simulink model "RobotResRateAlg"  (Simulink 7.8)
settings: Solver=ode45  StartTime=0.0  StopTime=simtime  RelTol=1e-3
values from neighbouring files (symbols this model uses):
  amp_C = 0.02    [projectCircle.m]
  freq_C = 2*pi/period    (= 0.1)    [projectCircle.m]
  Theta0 = fsolve(@inkinematic1,X0,optimset('Display','off'))    [projectCircle.m]
  Vx = 0    [projectCircle.m]
settings Model: Creator=carlossilvestre  LastModifiedBy=Administrator
settings DebuggingCC: SaveWithParameterizedLinksMsg=none  MultiTaskDSMMsg=warning  MultiTaskCondExecSysMsg=none  StrictBusMsg=None
settings RTWCC: IncludeERTFirstTime=on

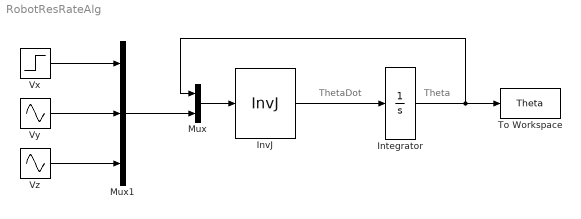
== system RobotResRateAlg ==
  note: ThetaDot
  note: Theta
  " Vz" : Sin  Amplitude=amp_C  Frequency=freq_C  Phase=pi/2  VectorParams1D=off
  Integrator : Integrator  InitialCondition=Theta0
  InvJ : MATLABFcn  MATLABFcn=InvJ  OutputDimensions=3
  Mux : Mux  Inputs=2
  Mux1 : Mux  Inputs=3
  To Workspace : ToWorkspace  VariableName=Theta  SampleTime=0.0342  SaveFormat=Array
  Vx : Step  Time=1000  Before=Vx  After=Vx
  Vy : Sin  Amplitude=amp_C  Frequency=freq_C  VectorParams1D=off
  wires:
  InvJ/1 -> Integrator/1
  Integrator/1 -> To Workspace/1, Mux/1
  Mux/1 -> InvJ/1
  Mux1/1 -> Mux/2
  Vx/1 -> Mux1/1
  Vy/1 -> Mux1/2
  " Vz"/1 -> Mux1/3
